simulink model "youbot_single_motor_analysis"  (R2017b)
settings: Solver=VariableStepAuto  StartTime=0.0  StopTime=5  RelTol=1e-4
values from neighbouring files (symbols this model uses):
  B_env = 1.8    [motor_model_kuka_youbot.m]    (also in motor_model_kuka_youbot2.m = 0.01)
  J = Jm + 1/(N^2)*(Jr + Jch)    (= 1.2077288055e-05)    [motor_model_kuka_youbot.m]    (also in motor_model_kuka_youbot2.m = 0.000181)
  K = k    (= 10)    [motor_model_kuka_youbot.m]    (also in motor_model_kuka_youbot2.m = i/1000)
  K_cur = Ki    (= 3.54813389234)    [Untitled.m]    (also in motor_model_kuka_youbot.m = 3000; motor_model_kuka_youbot2.m = 11.71875)
  K_env = 25    [motor_model_kuka_youbot.m]    (also in motor_model_kuka_youbot2.m = 1)
  Ke = 51.1e-3    (= 0.0511)    [motor_model_kuka_youbot.m]    (also in motor_model_kuka_youbot2.m = 1.10867309417)
  kf = R*Jm/L * 1e-6    (= 1.85e-11)    [motor_model_kuka_youbot.m]    (also in motor_model_kuka_youbot2.m = 0.000237684665227)
  Ki = 10^(11/20)    (= 3.54813389234)    [Untitled.m]    (also in motor_model_kuka_youbot.m = 1; motor_model_kuka_youbot2.m = j/1000)
  Ki_cur = Ki/Ti    (= 17740.6694617)    [Untitled.m]    (also in motor_model_kuka_youbot.m = 3000; motor_model_kuka_youbot2.m = 0.0114440917969)
  Kt = 51e-3    (= 0.051)    [motor_model_kuka_youbot.m]    (also in motor_model_kuka_youbot2.m = 0.0369)
  Kv = 200    [motor_model_kuka_youbot.m]    (also in motor_model_kuka_youbot2.m = 0.78125)
  L = 2.24    [motor_model_kuka_youbot.m]    (also in motor_model_kuka_youbot2.m = 0.000463)
  R = 4.48    [motor_model_kuka_youbot.m]    (also in motor_model_kuka_youbot2.m = 0.608)
libraries: simulink x1
settings Model: Creator=Vincent  LastModifiedBy=Vincent

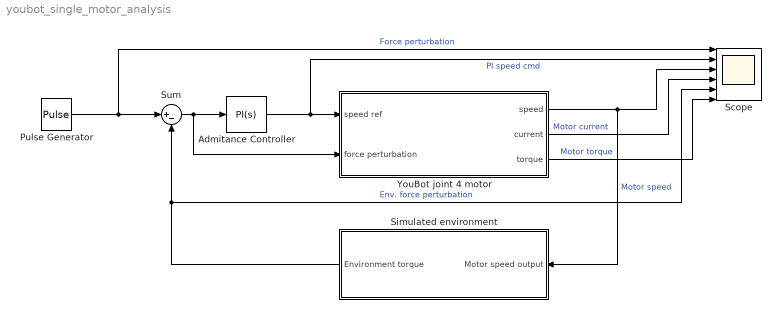
== system youbot_single_motor_analysis ==
  Admitance Controller : simulink/Continuous/PID Controller  Controller=PI  TimeDomain=Continuous-time  SampleTime=-1  IntegratorMethod=Forward Euler  FilterMethod=Forward Euler  Form=Parallel  UseFilter=on  ControllerParametersSource=internal  P=K  I=Ki  D=0  N=0  InitialConditionSource=internal  InitialConditionForIntegrator=0  InitialConditionForFilter=0  ExternalReset=none  LimitOutput=off  UpperSaturationLimit=inf  LowerSaturationLimit=-inf  LinearizeAsGain=on  AntiWindupMode=none  Kb=1  TrackingMode=off  Kt=1  PParamMin=[]  PParamMax=[]  IParamMin=[]  IParamMax=[]  DParamMin=[]  DParamMax=[]  NParamMin=[]  NParamMax=[]  KbParamMin=[]  KbParamMax=[]  KtParamMin=[]  KtParamMax=[]  POutMin=[]  POutMax=[]  IOutMin=[]  IOutMax=[]  DOutMin=[]  DOutMax=[]  NOutMin=[]  NOutMax=[]  KbOutMin=[]  KbOutMax=[]  KtOutMin=[]  KtOutMax=[]  IntegratorOutMin=[]  IntegratorOutMax=[]  FilterOutMin=[]  FilterOutMax=[]  SumOutMin=[]  SumOutMax=[]  SumI1OutMin=[]  SumI1OutMax=[]  SumI2OutMin=[]  SumI2OutMax=[]  SumI3OutMin=[]  SumI3OutMax=[]  SumDOutMin=[]  SumDOutMax=[]  SaturationOutMin=[]  SaturationOutMax=[]  IntegratorContinuousStateAttributes=''  IntegratorStateMustResolveToSignalObject=off  IntegratorRTWStateStorageClass=Auto  FilterContinuousStateAttributes=''  FilterStateMustResolveToSignalObject=off  FilterRTWStateStorageClass=Auto  DifferentiatorICPrevScaledInput=0  DifferentiatorOutMin=[]  DifferentiatorOutMax=[]  InitialConditionSetting=State (most efficient)  FilterDiffOutCoefMin=[]  FilterDiffOutCoefMax=[]  SumDenOutMin=[]  SumDenOutMax=[]  SumNumOutMin=[]  SumNumOutMax=[]  ReciprocalOutMin=[]  ReciprocalOutMax=[]  DivideOutMin=[]  DivideOutMax=[]  TunerSelectOption=Transfer Function Based (PID Tuner App)
  Pulse Generator : DiscretePulseGenerator  PulseType=Time based  PulseWidth=33
  Scope : Scope  NumInputPorts=6
  Simulated environment : Subsystem
  Sum : Sum  Inputs=|+-
  YouBot joint 4 motor : Subsystem
  wires:
  YouBot joint 4 motor/1(speed) -> Simulated environment/1(Motor speed output), Scope/3  "Motor speed"
  Admitance Controller/1 -> Scope/2, YouBot joint 4 motor/1(speed ref)  "PI speed cmd"
  Sum/1 -> YouBot joint 4 motor/2(force perturbation), Admitance Controller/1
  Pulse Generator/1 -> Sum/1, Scope/1  "Force perturbation"
  Simulated environment/1(Environment torque) -> Scope/5, Sum/2  "Env. force perturbation"
  YouBot joint 4 motor/2(current) -> Scope/4  "Motor current"
  YouBot joint 4 motor/3(torque) -> Scope/6  "Motor torque"

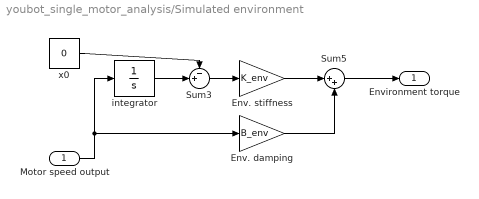
== system youbot_single_motor_analysis/Simulated environment ==
  Motor speed output : Inport
  Env. damping : Gain  Gain=B_env
  Env. stiffness : Gain  Gain=K_env
  Sum3 : Sum  Inputs=-+|
  Sum5 : Sum  Inputs=|++
  integrator : TransferFcn  Denominator=[1 0]
  x0 : Constant  Value=0
  Environment torque : Outport
  wires:
  integrator/1 -> Sum3/2
  x0/1 -> Sum3/1
  Sum3/1 -> Env. stiffness/1
  Sum5/1 -> Environment torque/1
  Env. damping/1 -> Sum5/2
  Env. stiffness/1 -> Sum5/1
  Motor speed output/1 -> Env. damping/1, integrator/1

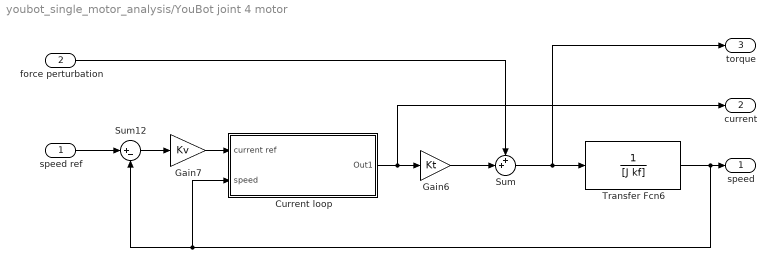
== system youbot_single_motor_analysis/YouBot joint 4 motor ==
  speed ref : Inport
  force perturbation : Inport  Port=2
  Current loop : Subsystem
  Gain6 : Gain  Gain=Kt
  Gain7 : Gain  Gain=Kv
  Sum : Sum  Inputs=++|
  Sum12 : Sum  Inputs=|+-
  Transfer Fcn6 : TransferFcn  Denominator=[J kf]
  speed : Outport
  current : Outport  Port=2
  torque : Outport  Port=3
  wires:
  speed ref/1 -> Sum12/1
  Sum12/1 -> Gain7/1
  Transfer Fcn6/1 -> speed/1, Current loop/2(speed), Sum12/2
  Gain7/1 -> Current loop/1(current ref)
  Current loop/1(Out1) -> current/1, Gain6/1
  Sum/1 -> torque/1, Transfer Fcn6/1
  force perturbation/1 -> Sum/1
  Gain6/1 -> Sum/2

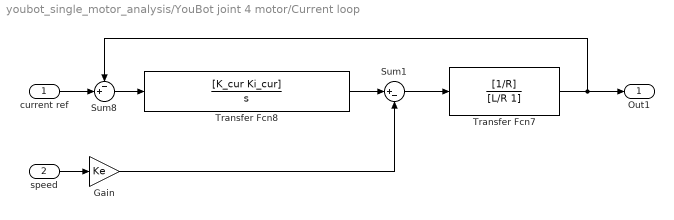
== system youbot_single_motor_analysis/YouBot joint 4 motor/Current loop ==
  current ref : Inport
  speed : Inport  Port=2
  Gain : Gain  Gain=Ke
  Sum1 : Sum  Inputs=|+-
  Sum8 : Sum  Inputs=-+|
  Transfer Fcn7 : TransferFcn  Numerator=[1/R]  Denominator=[L/R 1]
  Transfer Fcn8 : TransferFcn  Numerator=[K_cur Ki_cur]  Denominator=[1 0]
  Out1 : Outport
  wires:
  Sum8/1 -> Transfer Fcn8/1
  Transfer Fcn7/1 -> Out1/1, Sum8/1
  current ref/1 -> Sum8/2
  Transfer Fcn8/1 -> Sum1/1
  speed/1 -> Gain/1
  Gain/1 -> Sum1/2
  Sum1/1 -> Transfer Fcn7/1
